simulink model "Estim_DistCont_Fault2"  (R2018b)
settings: Solver=ode1  StartTime=0.0  StopTime=40000  FixedStep=1  RelTol=1e-3
InitFcn:
  | clearvars
  | modelcreation_simplified
  | addpath('C:\Users\u375749\Documents\Thesis\Codes\Linearization')
  | addpath('C:\Users\u375749\Documents\Thesis\Codes\MatlabPlant')
  | addpath('C:\Users\u375749\Documents\Thesis\Codes\ModelicaPlant\objects_inits')
  | addpath('C:\Users\u375749\Documents\Thesis\Codes\ModelicaPlant\matfiles')
  | addpath('C:\Users\u375749\Documents\Thesis\Codes\ModelicaPlant')
  | substitution_simplified
  | distributedControllers
  | delayT = 1*3;
  | delayh = 25*3;
  | hRatio = 1/3;
  | kfinit_simulink
  | rlsinit_simulink
  | faultinit_simulink
  | clear u
values from neighbouring files (symbols this model uses):
  fValues = 48    [faultcontrol3.mat]    (also in faultcontrol4.mat)
  npy = 2    [faultcontrol3.mat]    (also in faultcontrol4.mat)
  nr = 6    [faultcontrol3.mat]    (also in faultcontrol4.mat)
  sigma2p = 277777777.778    [faultcontrol3.mat]    (also in faultcontrol4.mat)
  sigma2T = 0.111111111111    [faultcontrol3.mat]    (also in faultcontrol4.mat)
  sigma2x = 1.11111111111e-05    [faultcontrol3.mat]    (also in faultcontrol4.mat)
  Ts = 1    [faultcontrol3.mat]    (also in faultcontrol4.mat)
  VValues = [0.0192 0.133 0.0001 0.00024]    [faultcontrol3.mat]    (also in faultcontrol4.mat)
undefined symbols (not defined in the file or in its folder): CoolProp, PI_C, PI_F, PI_GC, PI_HP, PI_LT, PI_MT, PI_RP, rls, x2q
libraries: simulink x2, FMIKit_blocks x1
settings Model: Creator=U370698  LastModifiedBy=U375749
settings DebuggingCC: LibraryContextMissingDiagnostic=none  UnderSpecifiedDimensionMsg=warning
settings SFSimCC: SimUseLocalCustomCode=off
settings RTWCC: RTWUseLocalCustomCode=off

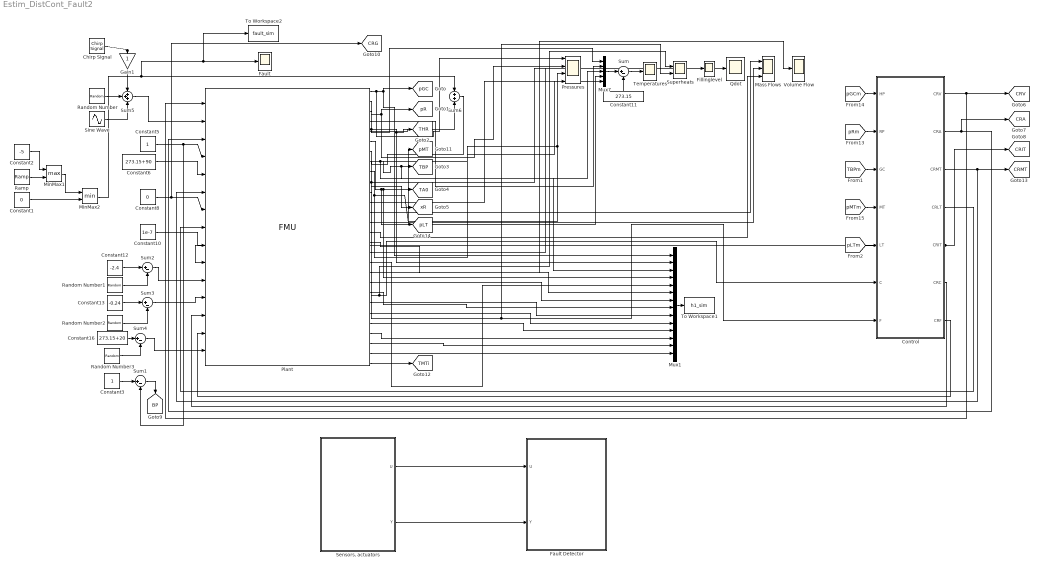
== system Estim_DistCont_Fault2 ==
  Chirp Signal : simulink/Sources/Chirp Signal  f1=2*pi/10000  T=30000  f2=2*pi*10/10000
  Constant1 : Constant  Value=0
  Constant10 : Constant  Value=1e-7
  Constant11 : Constant  Value=273.15
  Constant12 : Constant  Value=-2.4
  Constant13 : Constant  Value=-0.24
  Constant16 : Constant  Value=273.15+20
  Constant2 : Constant  Value=-5
  Constant3 : Constant
  Constant5 : Constant
  Constant6 : Constant  Value=273.15+90
  Constant8 : Constant  Value=0
  Control : Subsystem
  Fault : Scope
  Fault Detector : Subsystem
  Fillinglevel : Scope
  Gain1 : Gain
  Mass Flows : Scope  NumInputPorts=3
  MinMax1 : MinMax  Function=max  Inputs=2
  MinMax2 : MinMax  Inputs=2
  Mux1 : Mux  Inputs=14
  Mux7 : Mux  Inputs=5
  Plant : FMIKit_blocks/FMU  SFunctionModules=''
      settings: SourceProductName=FMI Kit
  Pressures : Scope  NumInputPorts=4
  Qdot : Scope
  Ramp : simulink/Sources/Ramp  slope=-1/10  start=20000  InitialOutput=0
  Random Number : RandomNumber  Variance=(1/10)^2/Ts  Seed=50  SampleTime=1
  Random Number1 : RandomNumber  Variance=(0.2/3)^2/Ts  Seed=51  SampleTime=1
  Random Number2 : RandomNumber  Variance=(0.02/3)^2/Ts  Seed=52  SampleTime=1
  Random Number3 : RandomNumber  Variance=(1/10)^2/Ts  Seed=53  SampleTime=1
  "Sensors, actuators" : Subsystem
  Sine Wave : Sin  Amplitude=10  Bias=273.15+20  Frequency=2*pi/10000  Phase=pi/2  SampleTime=0
  Sum{,1..4} (5 alike) : Sum  Inputs=|+-
  Sum5 : Sum  Inputs=+++
  Sum6 : Sum  Inputs=+|+
  Superheats : Scope  NumInputPorts=2
  Temperatures : Scope
  To Workspace1 : ToWorkspace  VariableName=h1_sim  SaveFormat=Structure With Time  SampleTime=-1
  To Workspace2 : ToWorkspace  VariableName=fault_sim  SaveFormat=Structure With Time  SampleTime=-1
  Volume Flow : Scope
  tag scope: BP=global, CRA=global, CRG=global, CRIT=global, CRMT=global, CRV=global, TA0=global, TBP=global, THR=global, TMTi=global, pGC=global, pLT=global, pMT=global, pR=global, xR=global
  wires:
  Sum5/1 -> Plant/2
  Constant5/1 -> Sum1/2, Plant/4
  Constant6/1 -> Plant/5
  Constant8/1 -> [CRG], Plant/7
  Constant10/1 -> Plant/9
  Plant/1 -> Mux1/1, [pGC], Pressures/1
  Constant11/1 -> Sum/2
  Sum/1 -> Temperatures/1
  Mux7/1 -> Sum/1
  Plant/3 -> Mux7/1, Mux1/2, [THR]
  Control/1(CRV) -> [CRV], Plant/1
  Control/2(CRA) -> [CRA], Plant/3
  Control/3(CRMT) -> Plant/6, [CRMT]
  Control/4(CRLT) -> Plant/8
  Control/6(CRC) -> Plant/13
  Control/7(CRF) -> Plant/14
  Plant/11 -> Control/7(F), Superheats/2
  Plant/10 -> Superheats/1, Control/6(C)
  Plant/9 -> [pLT], Pressures/4
  Plant/8 -> [pMT], Pressures/3
  Plant/7 -> [xR], Fillinglevel/1
  Plant/6 -> Mux1/4, [TA0], Mux7/4
  Plant/4 -> Mux7/2
  Sum6/1 -> Mux1/3, [TBP], Mux7/3
  Constant3/1 -> Sum1/1
  Sum1/1 -> [BP]
  Plant/2 -> [pR], Pressures/2
  Plant/13 -> Mass Flows/1
  Plant/14 -> Mass Flows/2
  Plant/15 -> Mass Flows/3
  Plant/17 -> Qdot/1
  Control/5(CRIT) -> [CRIT], Plant/10
  "Sensors, actuators"/1(U) -> Fault Detector/1(U)
  "Sensors, actuators"/2(Y) -> Fault Detector/2(Y)
  Mux1/1 -> To Workspace1/1
  Plant/12 -> Mux7/5
  Plant/27 -> Mux1/14
  Plant/26 -> Mux1/13
  Plant/25 -> Mux1/12
  Plant/24 -> Mux1/11
  Plant/23 -> Mux1/10
  Plant/22 -> Mux1/9
  Plant/21 -> Mux1/8
  Plant/20 -> Mux1/7
  Plant/19 -> Mux1/6
  Plant/18 -> Mux1/5
  Random Number/1 -> Sum5/2
  Constant12/1 -> Sum2/1
  Sum2/1 -> Plant/11
  Constant13/1 -> Sum3/1
  Sum3/1 -> Plant/12
  Random Number1/1 -> Sum2/2
  Random Number2/1 -> Sum3/2
  Constant16/1 -> Sum4/1
  Sum4/1 -> Plant/15
  Random Number3/1 -> Sum4/2
  Plant/5 -> Sum6/2
  Constant2/1 -> MinMax1/1
  Ramp/1 -> MinMax1/2
  MinMax2/1 -> To Workspace2/1, Fault/1, Sum6/1
  Chirp Signal/1 -> Gain1/1
  Gain1/1 -> Sum5/1
  Sine Wave/1 -> Sum5/3
  Constant1/1 -> MinMax2/2
  MinMax1/1 -> MinMax2/1
  Plant/28 -> [TMTi]
  Plant/16 -> Volume Flow/1
  [pGCm] -> Control/1(HP)
  [pRm] -> Control/2(RP)
  [TBPm] -> Control/3(GC)
  [pLTm] -> Control/5(LT)
  [pMTm] -> Control/4(MT)

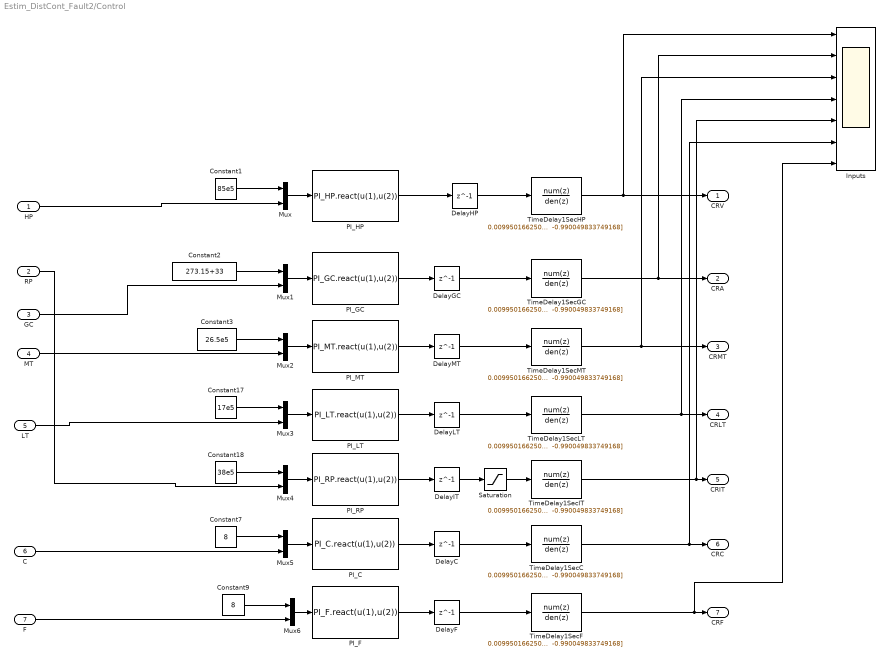
== system Estim_DistCont_Fault2/Control ==
  HP : Inport
  RP : Inport  Port=2
  GC : Inport  Port=3
  MT : Inport  Port=4
  LT : Inport  Port=5
  C : Inport  Port=6
  F : Inport  Port=7
  Constant1 : Constant  Value=85e5
  Constant17 : Constant  Value=17e5
  Constant18 : Constant  Value=38e5
  Constant2 : Constant  Value=273.15+33
  Constant3 : Constant  Value=26.5e5
  Constant7 : Constant  Value=8
  Constant9 : Constant  Value=8
  DelayC : Delay  DelayLength=1  InitialCondition=0.1
  DelayF : Delay  DelayLength=1  InitialCondition=0.04
  DelayGC : Delay  DelayLength=1  InitialCondition=0.625
  DelayHP : Delay  DelayLength=1  InitialCondition=0.25
  DelayIT : Delay  DelayLength=1  InitialCondition=0.45
  DelayLT : Delay  DelayLength=1  InitialCondition=0.3
  DelayMT : Delay  DelayLength=1  InitialCondition=0.3
  Inputs : Scope  NumInputPorts=7
  Mux{,1..6} (7 alike) : Mux  Inputs=2
  PI_C : MATLABFcn  MATLABFcn=PI_C.react(u(1),u(2))
  PI_F : MATLABFcn  MATLABFcn=PI_F.react(u(1),u(2))
  PI_GC : MATLABFcn  MATLABFcn=PI_GC.react(u(1),u(2))
  PI_HP : MATLABFcn  MATLABFcn=PI_HP.react(u(1),u(2))
  PI_LT : MATLABFcn  MATLABFcn=PI_LT.react(u(1),u(2))
  PI_MT : MATLABFcn  MATLABFcn=PI_MT.react(u(1),u(2))
  PI_RP : MATLABFcn  MATLABFcn=PI_RP.react(u(1),u(2))
  Saturation : Saturate  UpperLimit=0.7  LowerLimit=0
  TimeDelay1SecC : DiscreteTransferFcn  Numerator=0.009950166250832  Denominator="[1.000000000000000  -0.990049833749168]"
  TimeDelay1SecF : DiscreteTransferFcn  Numerator=0.009950166250832  Denominator="[1.000000000000000  -0.990049833749168]"
  TimeDelay1SecGC : DiscreteTransferFcn  Numerator=0.009950166250832  Denominator="[1.000000000000000  -0.990049833749168]"
  TimeDelay1SecHP : DiscreteTransferFcn  Numerator=0.009950166250832  Denominator="[1.000000000000000  -0.990049833749168]"
  TimeDelay1SecIT : DiscreteTransferFcn  Numerator=0.009950166250832  Denominator="[1.000000000000000  -0.990049833749168]"
  TimeDelay1SecLT : DiscreteTransferFcn  Numerator=0.009950166250832  Denominator="[1.000000000000000  -0.990049833749168]"
  TimeDelay1SecMT : DiscreteTransferFcn  Numerator=0.009950166250832  Denominator="[1.000000000000000  -0.990049833749168]"
  CRV : Outport
  CRA : Outport  Port=2
  CRMT : Outport  Port=3
  CRLT : Outport  Port=4
  CRIT : Outport  Port=5
  CRC : Outport  Port=6
  CRF : Outport  Port=7
  wires:
  MT/1 -> Mux2/2
  Mux3/1 -> PI_LT/1
  Mux4/1 -> PI_RP/1
  DelayHP/1 -> TimeDelay1SecHP/1
  Mux1/1 -> PI_GC/1
  DelayLT/1 -> TimeDelay1SecLT/1
  Constant2/1 -> Mux1/1
  Mux6/1 -> PI_F/1
  PI_HP/1 -> DelayHP/1
  Constant1/1 -> Mux/1
  PI_MT/1 -> DelayMT/1
  PI_LT/1 -> DelayLT/1
  PI_GC/1 -> DelayGC/1
  Mux2/1 -> PI_MT/1
  Constant18/1 -> Mux4/1
  Mux5/1 -> PI_C/1
  Constant7/1 -> Mux5/1
  Constant3/1 -> Mux2/1
  Constant9/1 -> Mux6/1
  PI_C/1 -> DelayC/1
  PI_F/1 -> DelayF/1
  PI_RP/1 -> DelayIT/1
  F/1 -> Mux6/2
  HP/1 -> Mux/2
  Constant17/1 -> Mux3/1
  Mux/1 -> PI_HP/1
  GC/1 -> Mux1/2
  LT/1 -> Mux3/2
  DelayC/1 -> TimeDelay1SecC/1
  DelayF/1 -> TimeDelay1SecF/1
  C/1 -> Mux5/2
  DelayGC/1 -> TimeDelay1SecGC/1
  DelayMT/1 -> TimeDelay1SecMT/1
  RP/1 -> Mux4/2
  TimeDelay1SecHP/1 -> Inputs/1, CRV/1
  TimeDelay1SecGC/1 -> Inputs/2, CRA/1
  TimeDelay1SecMT/1 -> Inputs/3, CRMT/1
  TimeDelay1SecLT/1 -> Inputs/4, CRLT/1
  TimeDelay1SecIT/1 -> Inputs/5, CRIT/1
  TimeDelay1SecC/1 -> Inputs/6, CRC/1
  TimeDelay1SecF/1 -> Inputs/7, CRF/1
  DelayIT/1 -> Saturation/1
  Saturation/1 -> TimeDelay1SecIT/1

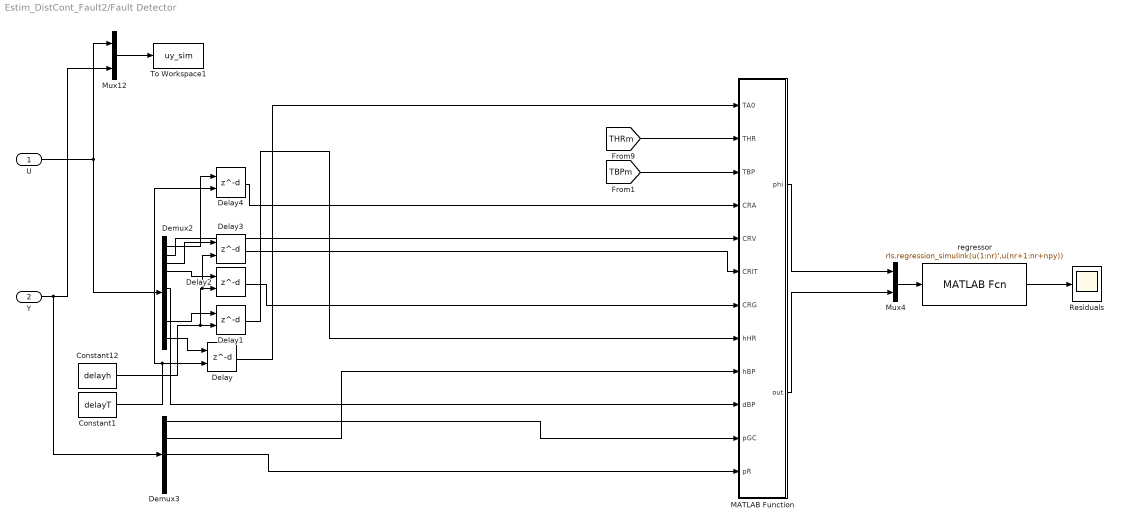
== system Estim_DistCont_Fault2/Fault Detector ==
  U : Inport
  Y : Inport  Port=2
  Constant1 : Constant  Value=delayT
  Constant12 : Constant  Value=delayh
  Delay : Delay  DelayLengthSource=Input port  DelayLength=delayh  InitialCondition=30+273
      settings: InputPortMap=u0,p1
  Delay1 : Delay  DelayLengthSource=Input port  DelayLength=delayh  InitialCondition=525e3
      settings: InputPortMap=u0,p1
  Delay2 : Delay  DelayLengthSource=Input port  DelayLength=delayh  InitialCondition=0.5
      settings: InputPortMap=u0,p1
  Delay3 : Delay  DelayLengthSource=Input port  DelayLength=delayh  InitialCondition=0.5
      settings: InputPortMap=u0,p1
  Delay4 : Delay  DelayLengthSource=Input port  DelayLength=delayh  InitialCondition=0.5
      settings: InputPortMap=u0,p1
  Demux2 : Demux  Outputs=12
  Demux3 : Demux  Outputs=5
  MATLAB Function : MATLAB Function  TreatAsAtomicUnit=on
  Mux12 : Mux  Inputs=2
  Mux4 : Mux  Inputs=2
  Residuals : Scope
  To Workspace1 : ToWorkspace  VariableName=uy_sim  SaveFormat=Structure With Time  SampleTime=-1
  regressor : MATLABFcn  MATLABFcn=rls.regression_simulink(u(1:nr)',u(nr+1:nr+npy))
  wires:
  Mux12/1 -> To Workspace1/1
  Y/1 -> Demux3/1, Mux12/2
  U/1 -> Demux2/1, Mux12/1
  Mux4/1 -> regressor/1
  regressor/1 -> Residuals/1
  MATLAB Function/2(out) -> Mux4/2
  MATLAB Function/1(phi) -> Mux4/1
  Constant1/1 -> Delay4/2, Delay/2
  Demux2/12 -> Delay/1
  Delay/1 -> MATLAB Function/1(TA0)
  Demux3/1 -> MATLAB Function/11(pGC)
  Demux2/10 -> Delay1/1
  Constant12/1 -> Delay3/2, Delay2/2, Delay1/2
  Demux2/4 -> Delay2/1
  Delay2/1 -> MATLAB Function/7(CRG)
  Demux2/3 -> Delay3/1
  Delay3/1 -> MATLAB Function/6(CRIT)
  Demux2/2 -> MATLAB Function/5(CRV)
  Demux2/1 -> Delay4/1
  Delay4/1 -> MATLAB Function/4(CRA)
  Demux3/3 -> MATLAB Function/12(pR)
  Demux2/6 -> MATLAB Function/10(dBP)
  Demux3/2 -> MATLAB Function/9(hBP)
  Delay1/1 -> MATLAB Function/8(hHR)
  [TBPm] -> MATLAB Function/3(TBP)
  [THRm] -> MATLAB Function/2(THR)

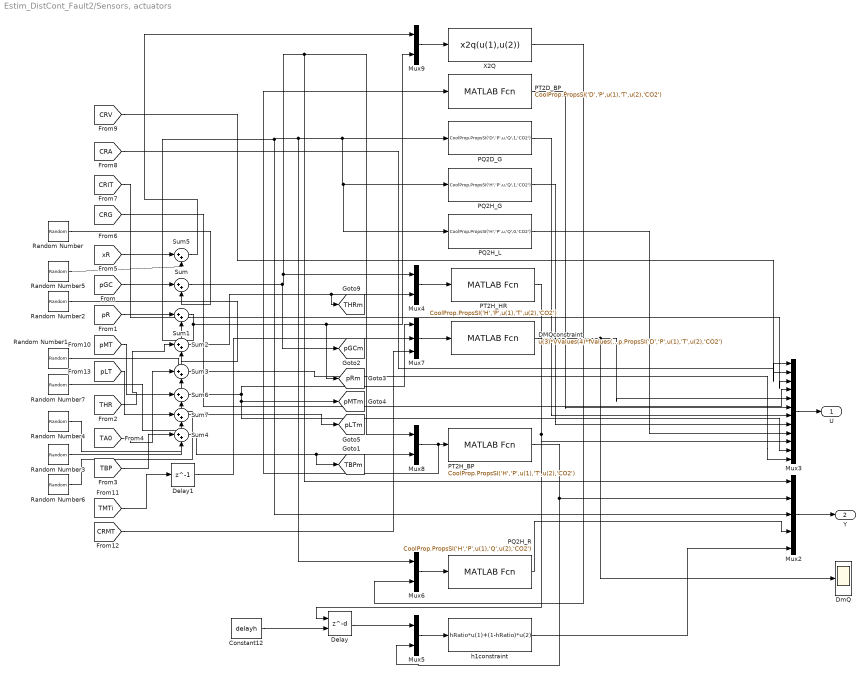
== system Estim_DistCont_Fault2/Sensors, actuators ==
  Constant12 : Constant  Value=delayh
  DMQconstraint : MATLABFcn  MATLABFcn=u(3)*VValues(4)*fValues(1)*CoolProp.PropsSI('D','P',u(1),'T',u(2),'CO2')
  Delay : Delay  DelayLengthSource=Input port  DelayLength=delayh  InitialCondition=525e3
      settings: InputPortMap=u0,p1
  Delay1 : Delay  DelayLength=1  InitialCondition=270
  DmQ : Scope
  Mux2 : Mux  Inputs=5
  Mux3 : Mux  Inputs=12
  Mux{4..6,8..9} (5 alike) : Mux  Inputs=2
  Mux7 : Mux  Inputs=3
  PQ2D_G : MATLABFcn  MATLABFcn=CoolProp.PropsSI('D','P',u,'Q',1,'CO2')
  PQ2H_G : MATLABFcn  MATLABFcn=CoolProp.PropsSI('H','P',u,'Q',1,'CO2')
  PQ2H_L : MATLABFcn  MATLABFcn=CoolProp.PropsSI('H','P',u,'Q',0,'CO2')
  PQ2H_R : MATLABFcn  MATLABFcn=CoolProp.PropsSI('H','P',u(1),'Q',u(2),'CO2')
  PT2D_BP : MATLABFcn  MATLABFcn=CoolProp.PropsSI('D','P',u(1),'T',u(2),'CO2')
  PT2H_BP : MATLABFcn  MATLABFcn=CoolProp.PropsSI('H','P',u(1),'T',u(2),'CO2')
  PT2H_HR : MATLABFcn  MATLABFcn=CoolProp.PropsSI('H','P',u(1),'T',u(2),'CO2')
  Random Number : RandomNumber  Variance=sigma2p/Ts  SampleTime=1
  Random Number1 : RandomNumber  Variance=sigma2T/Ts  Seed=10  SampleTime=1
  Random Number2 : RandomNumber  Variance=sigma2p/Ts  Seed=1  SampleTime=1
  Random Number3 : RandomNumber  Variance=sigma2T/Ts  Seed=12  SampleTime=1
  Random Number4 : RandomNumber  Variance=sigma2T/Ts  Seed=11  SampleTime=1
  Random Number5 : RandomNumber  Variance=sigma2x/Ts  Seed=21  SampleTime=1
  Random Number6 : RandomNumber  Variance=sigma2p/Ts  Seed=111  SampleTime=1
  Random Number7 : RandomNumber  Variance=sigma2T/Ts  Seed=10  SampleTime=112
  Sum{,1..7} (8 alike) : Sum  Inputs=|++
  X2Q : MATLABFcn  MATLABFcn=x2q(u(1),u(2))
  h1constraint : MATLABFcn  MATLABFcn=hRatio*u(1)+(1-hRatio)*u(2)
  U : Outport
  Y : Outport  Port=2
  tag scope: TBPm=global, THRm=global, pGCm=global, pLTm=global, pMTm=global, pRm=global
  wires:
  Sum1/1 -> Mux6/1, PQ2H_L/1, PQ2H_G/1, PQ2D_G/1, Mux2/3, [pRm], Mux9/2
  PT2H_HR/1 -> Delay/1, Mux3/10
  Sum/1 -> [pGCm], Mux2/1, Mux8/1, Mux4/1
  PQ2H_L/1 -> Mux3/9
  Sum5/1 -> Mux9/1
  [CRIT] -> Mux3/3
  PQ2H_R/1 -> Mux2/4
  PT2D_BP/1 -> Mux3/6
  DMQconstraint/1 -> DmQ/1, Mux3/5
  Mux9/1 -> X2Q/1
  [CRV] -> Mux3/2
  [CRA] -> Mux3/1
  PT2H_BP/1 -> Mux5/2, Mux2/2
  PQ2D_G/1 -> Mux3/7
  Mux8/1 -> PT2D_BP/1, PT2H_BP/1
  Mux4/1 -> PT2H_HR/1
  X2Q/1 -> Mux6/2
  PQ2H_G/1 -> Mux3/8
  Mux6/1 -> PQ2H_R/1
  Mux3/1 -> U/1
  Mux2/1 -> Y/1
  [pGC] -> Sum/1
  Random Number/1 -> Sum/2
  [pR] -> Sum1/1
  Random Number2/1 -> Sum1/2
  Sum2/1 -> [THRm], Mux4/2
  [THR] -> Sum2/1
  Random Number1/1 -> Sum2/2
  [TA0] -> Sum3/1
  Random Number3/1 -> Sum3/2
  [TBP] -> Sum4/1
  Random Number4/1 -> Sum4/2
  Random Number5/1 -> Sum5/2
  [xR] -> Sum5/1
  Mux5/1 -> h1constraint/1
  Sum4/1 -> [TBPm], Mux8/2
  Delay/1 -> Mux5/1
  h1constraint/1 -> Mux2/5
  Sum3/1 -> Mux3/12
  [CRG] -> Mux3/4
  Sum6/1 -> Mux3/11, [pMTm], Mux7/1
  Mux7/1 -> DMQconstraint/1
  [CRMT] -> Mux7/3
  [TMTi] -> Delay1/1
  Delay1/1 -> Mux7/2
  Constant12/1 -> Delay/2
  Random Number6/1 -> Sum6/2
  [pMT] -> Sum6/1
  Random Number7/1 -> Sum7/2
  [pLT] -> Sum7/1
  Sum7/1 -> [pLTm]

== matlab function Estim_DistCont_Fault2/Fault Detector/MATLAB Function ==
  data: TA0 input; phi output; THR input; TBP input; out output; CRA input; CRV input; CRIT input; CRG input; hHR input; hBP input; dBP input; pGC input; pR input
function [phi,out] = fcn(TA0,THR,TBP,CRA,CRV,CRIT,CRG,hHR,hBP,dBP,pGC,pR)


DmV = CRV*0.8*3e-5*sqrt(dBP*(pGC - pR));
DQ = DmV*(hHR - hBP);
phi = [1; CRA; CRV; TA0-273; CRIT; CRG; THR-273];
out = [DQ TBP];
